simulink model "Leader"  (R2024b)
settings: Solver=ode4  StartTime=0  StopTime=100  FixedStep=0.001  RelTol=1e-3
undefined symbols (not defined in the file or in its folder): DiscIntNeverNeededParam
libraries: simulink x22, vrlib x1
(part 1 of 4)
settings Model: Creator=moham  LastModifiedBy=Omar
settings SolverCC: AlgebraicLoopSolver=TrustRegion
settings DataIOCC: ReturnWorkspaceOutputs=off
settings OptimizationCC: ReuseModelBlockBuffer=off
settings DebuggingCC: UnconnectedInputMsg=warning  UnconnectedOutputMsg=warning  UnconnectedLineMsg=warning  ArithmeticOperatorsInVariantConditions=warning
settings ModelReferenceCC: EnableRefExpFcnMdlSchedulingChecks=on
settings SFSimCC: SimUseLocalCustomCode=off  CustomCodeUndefinedFunction=UseInterfaceOnly
settings RTWCC: RTWUseLocalCustomCode=off  GPUComputeCapability=3.5

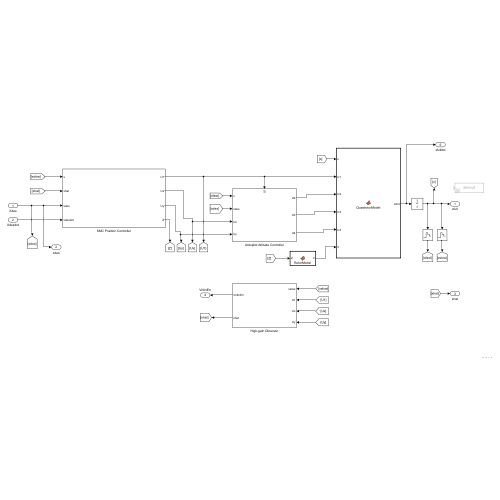
[thumbnail: Simulink's stored preview of the top-level diagram]
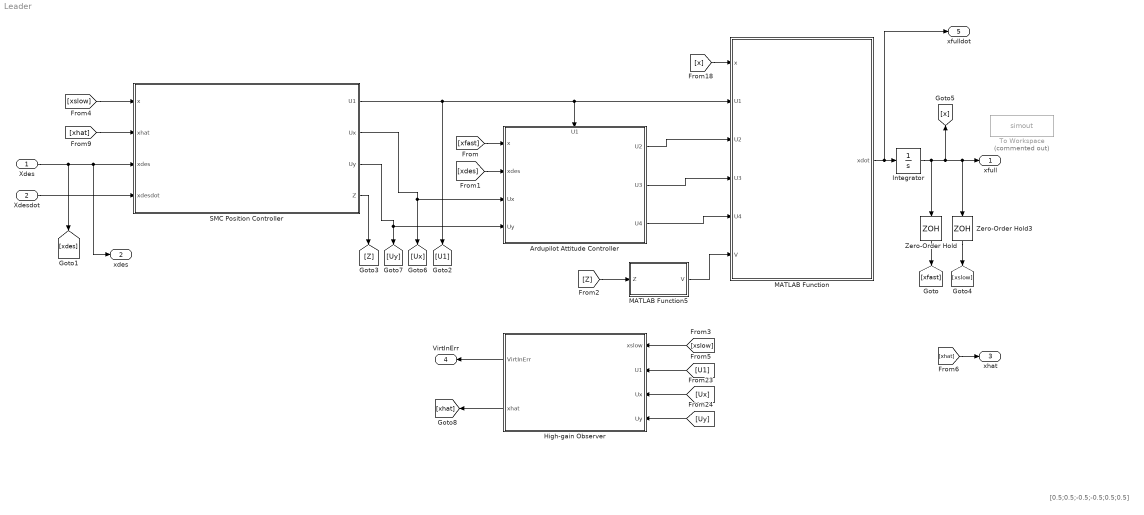
== system Leader ==
  note: [0.5;0.5;-0.5;-0.5;0.5;0.5]
  Xdes : Inport
  Xdesdot : Inport  Port=2  PortDimensions=12
  Ardupilot Attitude Controller : Subsystem
      settings: PortSchema="{\"entries\":[{\"content\":{\"sides\":[{\"content\":{\"connectorIds\":[\"In1\",\"In2\",\"In3\",\"In4\"]},\"type\":\"ConnectorPlacement.EquallySpacedRectSide\",\"uuid\":\"bad7bc7b-c5aa-4aa4-9de0-2ec046c1796f\"},{\"content\":{\"connectorIds\":[\"Out1\",\"Out2\",\"Out3\"],\"side\":\"RIGHT\"},\"type\":\"ConnectorPlacement.EquallySpacedRectSide\",\"uuid\":\"8bce01b0-d4dd-493d-8a35-b9dc86decf14\"},{\"content\":{\"connectorIds\":[\"In5\"],\"side\":\"TOP\"},\"type\":\"ConnectorPlacement.EquallySpacedRectSide\",\"uuid\":\"7d374ae2-e477-4008-a0c5-b6f4f89ed51f\"}]},\"type\":\"ConnectorPlacement.EquallySpacedConnector\",\"uuid\":\"7f04a3db-e2da-43c2-a92f-32b1947c5415\"}],\"packageUris\":[\"http://schema.mathworks.com/mf0/Connector/19700101\"],\"version\":\"1.0\"}"
  High-gain Observer : Subsystem
  Integrator : Integrator  InitialCondition=[0;0;0;0;0;0;0;0;0;0;0;0;0;0;0;0]
  MATLAB Function : MATLAB Function  TreatAsAtomicUnit=on
  MATLAB Function5 : MATLAB Function  TreatAsAtomicUnit=on
  SMC Position Controller : Subsystem
  To Workspace : ToWorkspace  Commented=on  VariableName=simout  SampleTime=-1
  Zero-Order Hold : ZeroOrderHold  SampleTime=0.01
  Zero-Order Hold3 : ZeroOrderHold  SampleTime=0.02
  xfull : Outport  VectorParamsAs1DForOutWhenUnconnected=off
  xdes : Outport  Port=2  VectorParamsAs1DForOutWhenUnconnected=off
  xhat : Outport  Port=3
  VirtInErr : Outport  Port=4
  xfulldot : Outport  Port=5
  wires:
  MATLAB Function5/1(V) -> MATLAB Function/6(V)
  MATLAB Function/1(xdot) -> xfulldot/1, Integrator/1
  Integrator/1 -> Zero-Order Hold3/1, xfull/1, [x], Zero-Order Hold/1
  Ardupilot Attitude Controller/1(U2) -> MATLAB Function/3(U2)
  Ardupilot Attitude Controller/2(U3) -> MATLAB Function/4(U3)
  Ardupilot Attitude Controller/3(U4) -> MATLAB Function/5(U4)
  [xdes] -> Ardupilot Attitude Controller/2(xdes)
  [x] -> MATLAB Function/1(x)
  [xslow] -> SMC Position Controller/1(x)
  [xhat] -> SMC Position Controller/2(xhat)
  Xdes/1 -> SMC Position Controller/3(xdes), xdes/1, [xdes]
  Xdesdot/1 -> SMC Position Controller/4(xdesdot)
  SMC Position Controller/1(U1) -> Ardupilot Attitude Controller/5(U1), MATLAB Function/2(U1), [U1]
  SMC Position Controller/2(Ux) -> [Ux], Ardupilot Attitude Controller/3(Ux)
  SMC Position Controller/3(Uy) -> Ardupilot Attitude Controller/4(Uy), [Uy]
  SMC Position Controller/4(Z) -> [Z]
  [Z] -> MATLAB Function5/1(Z)
  Zero-Order Hold/1 -> [xfast]
  Zero-Order Hold3/1 -> [xslow]
  [xhat] -> xhat/1
  [xfast] -> Ardupilot Attitude Controller/1(x)
  [U1] -> High-gain Observer/2(U1)
  [Ux] -> High-gain Observer/3(Ux)
  [Uy] -> High-gain Observer/4(Uy)
  [xslow] -> High-gain Observer/1(xslow)
  High-gain Observer/2(xhat) -> [xhat]
  High-gain Observer/1(VirtInErr) -> VirtInErr/1

== system Leader/Ardupilot Attitude Controller ==
  note: Get Desired Attitude
  note: Forward Desired Yaw and Convert: Virtual
      | Inputs --> Desired Roll and Pitch angles
  note: Rate Controller
  note: Attitude Controller
  x : Inport
  xdes : Inport  Port=2
  Ux : Inport  Port=3
  Uy : Inport  Port=4
  U1 : Inport  Port=5
  Attitude Controller : Subsystem
      settings: PortSchema="{\"entries\":[{\"content\":{\"sides\":[{\"content\":{\"connectorIds\":[\"In1\",\"In2\",\"In3\",\"In4\"]},\"type\":\"ConnectorPlacement.EquallySpacedRectSide\",\"uuid\":\"ec7fb444-4fa0-4c75-9921-499ce0d65b3a\"},{\"content\":{\"connectorIds\":[\"Out1\",\"Out2\",\"Out3\",\"Out4\"],\"side\":\"RIGHT\"},\"type\":\"ConnectorPlacement.EquallySpacedRectSide\",\"uuid\":\"c514eb8b-c928-4fdc-8f94-1e92d461987d\"},{\"content\":{\"connectorIds\":[],\"side\":\"TOP\"},\"type\":\"ConnectorPlacement.EquallySpacedRectSide\",\"uuid\":\"c9522f68-fcfa-40bc-963d-dafc938ce27d\"},{\"content\":{\"connectorIds\":[\"In5\",\"In6\",\"In7\"],\"side\":\"BOTTOM\"},\"type\":\"ConnectorPlacement.EquallySpacedRectSide\",\"uuid\":\"bc7d5f1e-3200-477e-805f-b3259f0159e2\"}]},\"type\":\"ConnectorPlacement.EquallySpacedConnector\",\"uuid\":\"993ff006-2c19-4b52-a807-2d91f7e143b6\"}],\"packageUris\":[\"http://schema.mathworks.com/mf0/Connector/19700101\"],\"version\":\"1.0\"}"
  Demux : Demux  Outputs=3
  Divide : Product  Inputs=*/
  MATLAB Function : MATLAB Function  TreatAsAtomicUnit=on
  MATLAB Function4 : MATLAB Function
  Max Thrust : Constant  Value=39
  Rate Controller : Subsystem
      settings: PortSchema="{\"entries\":[{\"content\":{\"sides\":[{\"content\":{\"connectorIds\":[\"In1\",\"In2\",\"In3\"]},\"type\":\"ConnectorPlacement.EquallySpacedRectSide\",\"uuid\":\"8a701ca7-ce38-496e-9f89-73a8426d5a34\"},{\"content\":{\"connectorIds\":[\"Out1\",\"Out2\",\"Out3\"],\"side\":\"RIGHT\"},\"type\":\"ConnectorPlacement.EquallySpacedRectSide\",\"uuid\":\"363a0e2e-6acc-4f21-9121-ba7c8748d9b4\"},{\"content\":{\"connectorIds\":[],\"side\":\"TOP\"},\"type\":\"ConnectorPlacement.EquallySpacedRectSide\",\"uuid\":\"4d7a2121-90ee-4dbe-91e3-b86ad0b96fd9\"},{\"content\":{\"connectorIds\":[\"In4\",\"In5\",\"In6\"],\"side\":\"BOTTOM\"},\"type\":\"ConnectorPlacement.EquallySpacedRectSide\",\"uuid\":\"495eef18-c57e-4f49-baa4-5500712935f3\"}]},\"type\":\"ConnectorPlacement.EquallySpacedConnector\",\"uuid\":\"9c8722b4-18d5-4647-94e4-af7446d3f664\"}],\"packageUris\":[\"http://schema.mathworks.com/mf0/Connector/19700101\"],\"version\":\"1.0\"}"
  Scope3 : Scope  NumInputPorts=3
  Selector2 : Selector  InputPortWidth=16  IndexOptions=Index vector (dialog)  Indices=[1 3 5]  OutputSizes=1
  Selector3 : Selector  InputPortWidth=16  IndexOptions=Index vector (dialog)  Indices=[2 4 6]  OutputSizes=1
  Terminator : Terminator
  U2 : Outport  VectorParamsAs1DForOutWhenUnconnected=off
  U3 : Outport  Port=2  VectorParamsAs1DForOutWhenUnconnected=off
  U4 : Outport  Port=3  VectorParamsAs1DForOutWhenUnconnected=off
  wires:
  xdes/1 -> MATLAB Function4/2(xdes)
  Attitude Controller/1(rollRateTar) -> Rate Controller/1(rollRateDes)  "rollRateTar"
  Attitude Controller/4(feedforwardScaler) -> Terminator/1
  Attitude Controller/2(pitchRateTar) -> Rate Controller/2(pitchRateDes)  "pitchRateTar"
  Attitude Controller/3(yawRateTar) -> Rate Controller/3(yawRateDes)  "yawRateTar"
  x/1 -> MATLAB Function4/1(x), [x]
  Max Thrust/1 -> Divide/2
  Divide/1 -> [throttle]
  [throttle] -> Attitude Controller/1(throttle)
  MATLAB Function4/1(phi_des) -> Attitude Controller/2(rollAngDes)
  MATLAB Function4/2(theta_des) -> Attitude Controller/3(pitchAngDes)
  MATLAB Function4/3(psidot_des) -> Attitude Controller/4(yawRateDes)
  [x] -> Selector3/1, Selector2/1
  Selector2/1 -> [eulerAct]
  Selector3/1 -> [ratesAct]
  [eulerAct] -> MATLAB Function/1(euler), Attitude Controller/5(eulerAngleAct)
  MATLAB Function/1(q) -> Attitude Controller/6(attitudeBodyAct)
  [ratesAct] -> Attitude Controller/7(angRatesBf)
  Demux/1 -> Rate Controller/4(rollRateAct)
  Demux/2 -> Rate Controller/5(pitchRateAct)
  Demux/3 -> Rate Controller/6(yawRateAct)
  Rate Controller/1(rollRateCtrlOut) -> U2/1, Scope3/1
  Rate Controller/2(pitchRateCtrlOut) -> Scope3/2, U3/1
  Rate Controller/3(yawRateCtrlOut) -> Scope3/3, U4/1
  Ux/1 -> MATLAB Function4/3(Ux)
  Uy/1 -> MATLAB Function4/4(Uy)
  U1/1 -> Divide/1
  [ratesAct] -> Demux/1

== system Leader/High-gain Observer ==
  note: Inputs
  note: Trapezoidal Integration for
      | Estimation Errors in Z
  note: High-gain Observer
      | (Updating State Estimates)
  note: Outputs
  xslow : Inport
  U1 : Inport  Port=2
  Ux : Inport  Port=3
  Uy : Inport  Port=4
  Discrete-Time Integrator : DiscreteIntegrator  SampleTime=-1  ICPrevOutput=DiscIntNeverNeededParam  ICPrevScaledInput=DiscIntNeverNeededParam
  Integrator1 : Integrator  InitialCondition=[0.0;0.0;-1;0;0;0]
  MATLAB Function2 : MATLAB Function  TreatAsAtomicUnit=on
  Mux1 : Mux  Inputs=2
  Selector : Selector  InputPortWidth=16  IndexOptions=Index vector (dialog)  Indices=[11]  OutputSizes=1
  Selector1 : Selector  InputPortWidth=6  IndexOptions=Index vector (dialog)  Indices=[5]  OutputSizes=1
  Sum : Sum  Inputs=|+-
  Sum1 : Sum  Inputs=|+-
  Zero-Order Hold2 : ZeroOrderHold  SampleTime=0.02
  VirtInErr : Outport
  xhat : Outport  Port=2
  wires:
  Zero-Order Hold2/1 -> [xhat]
  Mux1/1 -> Sum1/2
  [xslow] -> MATLAB Function2/1(x)
  MATLAB Function2/2(UxUyact) -> Sum1/1
  [xhat] -> Selector1/1
  MATLAB Function2/1(xhatdot) -> Integrator1/1
  [Ux] -> Mux1/1
  [U1] -> MATLAB Function2/4(U1)
  Integrator1/1 -> Zero-Order Hold2/1
  Sum1/1 -> VirtInErr/1
  [Uy] -> Mux1/2
  Sum/1 -> Discrete-Time Integrator/1
  [xhat] -> MATLAB Function2/3(xhat)
  Selector/1 -> Sum/1
  Selector1/1 -> Sum/2
  U1/1 -> [U1]
  Ux/1 -> [Ux]
  Uy/1 -> [Uy]
  xslow/1 -> [xslow]
  [xslow] -> Selector/1
  Discrete-Time Integrator/1 -> MATLAB Function2/2(zintg)
  [xhat] -> xhat/1

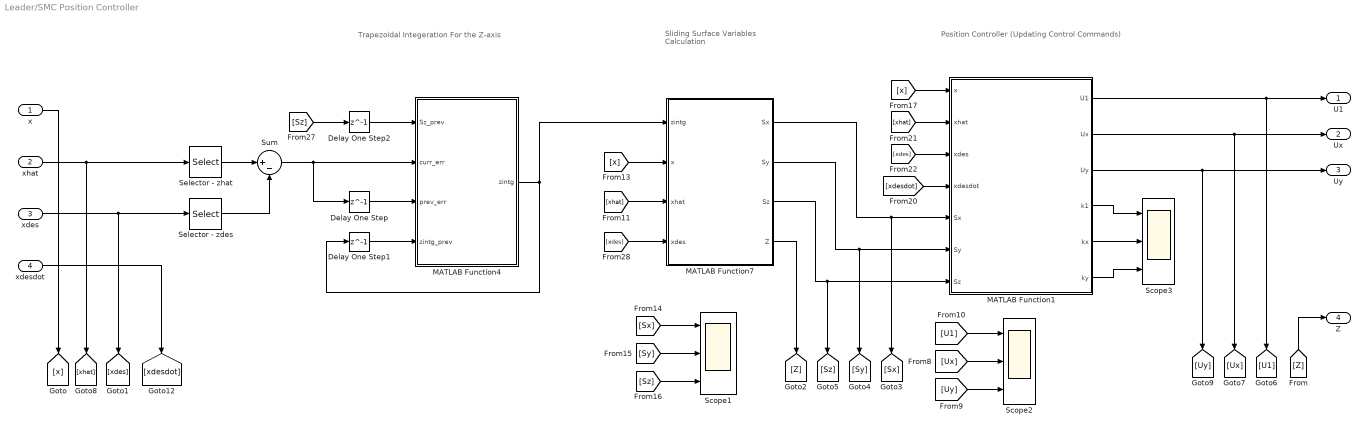
== system Leader/SMC Position Controller ==
  note: Sliding Surface
      | Variables Calculation
  note: Trapezoidal Integeration
      | For the Z-axis
  note: Position Controller
      | (Updating Control Commands)
  x : Inport
  xhat : Inport  Port=2
  xdes : Inport  Port=3
  xdesdot : Inport  Port=4
  Delay One Step : Delay  DelayLength=1
  Delay One Step1 : Delay  DelayLength=1
  Delay One Step2 : Delay  DelayLength=1
  MATLAB Function1 : MATLAB Function  TreatAsAtomicUnit=on
  MATLAB Function4 : MATLAB Function  TreatAsAtomicUnit=on
  MATLAB Function7 : MATLAB Function  TreatAsAtomicUnit=on
  Scope1 : Scope  NumInputPorts=3
  Scope2 : Scope  NumInputPorts=3
  Scope3 : Scope  NumInputPorts=3
  Selector - zdes : Selector  InputPortWidth=12  IndexOptions=Index vector (dialog)  Indices=[11]  OutputSizes=1
  Selector - zhat : Selector  InputPortWidth=6  IndexOptions=Index vector (dialog)  Indices=[5]  OutputSizes=1
  Sum : Sum  Inputs=|+-
  U1 : Outport
  Ux : Outport  Port=2
  Uy : Outport  Port=3
  Z : Outport  Port=4
  wires:
  [Sz] -> Delay One Step2/1
  Selector - zhat/1 -> Sum/1
  Sum/1 -> Delay One Step/1, MATLAB Function4/2(curr_err)
  Delay One Step2/1 -> MATLAB Function4/1(Sz_prev)
  Delay One Step1/1 -> MATLAB Function4/4(zintg_prev)
  MATLAB Function4/1(zintg) -> MATLAB Function7/1(zintg), Delay One Step1/1
  Selector - zdes/1 -> Sum/2
  Delay One Step/1 -> MATLAB Function4/3(prev_err)
  xhat/1 -> [xhat], Selector - zhat/1
  xdes/1 -> [xdes], Selector - zdes/1
  [xdes] -> MATLAB Function7/4(xdes)
  [xhat] -> MATLAB Function7/3(xhat)
  [x] -> MATLAB Function7/2(x)
  x/1 -> [x]
  xdesdot/1 -> [xdesdot]
  [xdesdot] -> MATLAB Function1/4(xdesdot)
  [x] -> MATLAB Function1/1(x)
  [xhat] -> MATLAB Function1/2(xhat)
  [xdes] -> MATLAB Function1/3(xdes)
  MATLAB Function7/1(Sx) -> [Sx], MATLAB Function1/5(Sx)
  MATLAB Function7/2(Sy) -> [Sy], MATLAB Function1/6(Sy)
  MATLAB Function7/3(Sz) -> [Sz], MATLAB Function1/7(Sz)
  MATLAB Function7/4(Z) -> [Z]
  MATLAB Function1/1(U1) -> [U1], U1/1
  MATLAB Function1/2(Ux) -> [Ux], Ux/1
  MATLAB Function1/3(Uy) -> [Uy], Uy/1
  [Z] -> Z/1
  [Sz] -> Scope1/3
  [U1] -> Scope2/1
  [Sy] -> Scope1/2
  [Sx] -> Scope1/1
  [Ux] -> Scope2/2
  [Uy] -> Scope2/3
  MATLAB Function1/4(k1) -> Scope3/1
  MATLAB Function1/5(kx) -> Scope3/2
  MATLAB Function1/6(ky) -> Scope3/3

== system Leader/Ardupilot Attitude Controller/Attitude Controller ==
  note: input_euler_angle_roll_pitch_euler_rate_yaw() & attitude_controller_run_quat()
      | Calculation of target euler rates and angles and angular velocities
  note: Sponsored by IAV GmbH
  throttle : Inport
  rollAngDes : Inport  Port=2
  pitchAngDes : Inport  Port=3
  yawRateDes : Inport  Port=4
  eulerAngleAct : Inport  Port=5
  attitudeBodyAct : Inport  Port=6
  angRatesBf : Inport  Port=7
  Demux : Demux  Outputs=3
  input_euler_angle_roll_pitch_euler_rate_yaw() : Subsystem
  rollRateTar : Outport
  pitchRateTar : Outport  Port=2
  yawRateTar : Outport  Port=3
  feedforwardScaler : Outport  Port=4
  wires:
  attitudeBodyAct/1 -> input_euler_angle_roll_pitch_euler_rate_yaw()/6(attitudeBodyAct)
  angRatesBf/1 -> input_euler_angle_roll_pitch_euler_rate_yaw()/7(angRatesBf)
  Demux/2 -> pitchRateTar/1
  Demux/1 -> rollRateTar/1
  Demux/3 -> yawRateTar/1
  input_euler_angle_roll_pitch_euler_rate_yaw()/1(angVelBodyTarget) -> Demux/1  "angVelBody"
  input_euler_angle_roll_pitch_euler_rate_yaw()/2(feedforwardScaler) -> feedforwardScaler/1
  eulerAngleAct/1 -> input_euler_angle_roll_pitch_euler_rate_yaw()/5(eulerAngleAct)
  throttle/1 -> input_euler_angle_roll_pitch_euler_rate_yaw()/1(throttle)
  rollAngDes/1 -> input_euler_angle_roll_pitch_euler_rate_yaw()/2(rollAngDes)
  pitchAngDes/1 -> input_euler_angle_roll_pitch_euler_rate_yaw()/3(pitchAngDes)
  yawRateDes/1 -> input_euler_angle_roll_pitch_euler_rate_yaw()/4(yawRateDes)

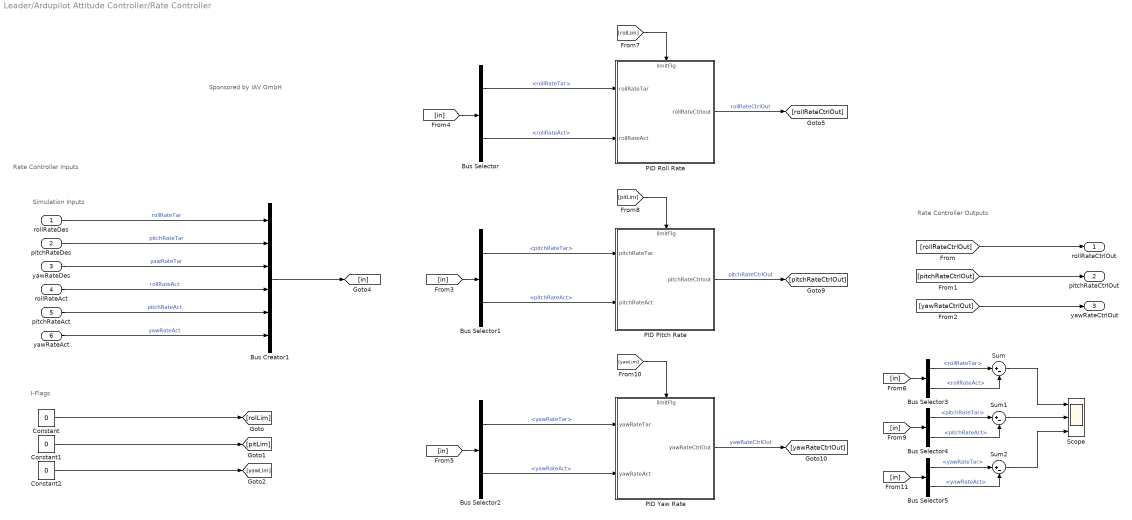
== system Leader/Ardupilot Attitude Controller/Rate Controller ==
  note: I-Flags
  note: Rate Controller Inputs
  note: Rate Controller Outputs
  note: Simulation Inputs
  note: Sponsored by IAV GmbH
  rollRateDes : Inport
  pitchRateDes : Inport  Port=2
  yawRateDes : Inport  Port=3
  rollRateAct : Inport  Port=4
  pitchRateAct : Inport  Port=5
  yawRateAct : Inport  Port=6
  Bus Creator1 : BusCreator  Inputs=6
  Bus Selector : BusSelector  OutputSignals=rollRateTar,rollRateAct
  Bus Selector1 : BusSelector  OutputSignals=pitchRateTar,pitchRateAct
  Bus Selector2 : BusSelector  OutputSignals=yawRateTar,yawRateAct
  Bus Selector3 : BusSelector  OutputSignals=rollRateTar,rollRateAct
  Bus Selector4 : BusSelector  OutputSignals=pitchRateTar,pitchRateAct
  Bus Selector5 : BusSelector  OutputSignals=yawRateTar,yawRateAct
  Constant : Constant  Value=0
  Constant1 : Constant  Value=0
  Constant2 : Constant  Value=0
  PID Pitch Rate : Subsystem
      settings: PortSchema="{\"entries\":[{\"content\":{\"sides\":[{\"content\":{\"connectorIds\":[\"In1\",\"In2\"]},\"type\":\"ConnectorPlacement.EquallySpacedRectSide\",\"uuid\":\"c953bf57-30fb-4394-aa81-6fda736b57a6\"},{\"content\":{\"connectorIds\":[\"Out1\"],\"side\":\"RIGHT\"},\"type\":\"ConnectorPlacement.EquallySpacedRectSide\",\"uuid\":\"3c7ad81e-0863-4191-b28a-a9c07f820a0a\"},{\"content\":{\"connectorIds\":[\"In3\"],\"side\":\"TOP\"},\"type\":\"ConnectorPlacement.EquallySpacedRectSide\",\"uuid\":\"d279fa4b-d6e6-48af-a4f1-9d8595a6d70c\"}]},\"type\":\"ConnectorPlacement.EquallySpacedConnector\",\"uuid\":\"40596868-642f-4372-b8bb-11353e7a9cdb\"}],\"packageUris\":[\"http://schema.mathworks.com/mf0/Connector/19700101\"],\"version\":\"1.0\"}"
  PID Roll Rate : Subsystem
      settings: PortSchema="{\"entries\":[{\"content\":{\"sides\":[{\"content\":{\"connectorIds\":[\"In1\",\"In2\"]},\"type\":\"ConnectorPlacement.EquallySpacedRectSide\",\"uuid\":\"ccc00f8c-3713-4b46-9b2d-67fda6f44eb9\"},{\"content\":{\"connectorIds\":[\"Out1\"],\"side\":\"RIGHT\"},\"type\":\"ConnectorPlacement.EquallySpacedRectSide\",\"uuid\":\"24a560ef-4b0d-44d4-b17e-8cb38dfcb6b4\"},{\"content\":{\"connectorIds\":[\"In3\"],\"side\":\"TOP\"},\"type\":\"ConnectorPlacement.EquallySpacedRectSide\",\"uuid\":\"cd43f1cb-999b-4e44-9f37-57514624398c\"}]},\"type\":\"ConnectorPlacement.EquallySpacedConnector\",\"uuid\":\"35b9a70d-95bd-44f6-87a8-68a113e8ff9b\"}],\"packageUris\":[\"http://schema.mathworks.com/mf0/Connector/19700101\"],\"version\":\"1.0\"}"
  PID Yaw Rate : Subsystem
      settings: PortSchema="{\"entries\":[{\"content\":{\"sides\":[{\"content\":{\"connectorIds\":[\"In1\",\"In2\"]},\"type\":\"ConnectorPlacement.EquallySpacedRectSide\",\"uuid\":\"e641bc52-3ba8-4abf-91e5-f3e8f1d63eab\"},{\"content\":{\"connectorIds\":[\"Out1\"],\"side\":\"RIGHT\"},\"type\":\"ConnectorPlacement.EquallySpacedRectSide\",\"uuid\":\"7d55638e-b8f2-47ab-a11f-a4e45a3d6a7b\"},{\"content\":{\"connectorIds\":[\"In3\"],\"side\":\"TOP\"},\"type\":\"ConnectorPlacement.EquallySpacedRectSide\",\"uuid\":\"6a487507-9fdf-4d3e-b86b-b3f94c6d2850\"}]},\"type\":\"ConnectorPlacement.EquallySpacedConnector\",\"uuid\":\"38d20622-e21d-450d-bf23-0a2964a9c200\"}],\"packageUris\":[\"http://schema.mathworks.com/mf0/Connector/19700101\"],\"version\":\"1.0\"}"
  Scope : Scope  NumInputPorts=3
  Sum : Sum  Inputs=|+-
  Sum1 : Sum  Inputs=|+-
  Sum2 : Sum  Inputs=|+-
  rollRateCtrlOut : Outport
  pitchRateCtrlOut : Outport  Port=2
  yawRateCtrlOut : Outport  Port=3
  wires:
  PID Yaw Rate/1(yawRateCtrlOut) -> [yawRateCtrlOut]  "yawRateCtrlOut"
  Bus Selector/1 -> PID Roll Rate/1(rollRateTar)  "<rollRateTar>"
  Bus Selector/2 -> PID Roll Rate/2(rollRateAct)  "<rollRateAct>"
  Bus Selector2/1 -> PID Yaw Rate/1(yawRateTar)  "<yawRateTar>"
  PID Pitch Rate/1(pitchRateCtrlout) -> [pitchRateCtrlOut]  "pitchRateCtrlOut"
  Bus Selector2/2 -> PID Yaw Rate/2(yawRateAct)  "<yawRateAct>"
  PID Roll Rate/1(rollRateCtrlout) -> [rollRateCtrlOut]  "rollRateCtrlOut"
  [rollRateCtrlOut] -> rollRateCtrlOut/1
  [pitchRateCtrlOut] -> pitchRateCtrlOut/1
  [yawRateCtrlOut] -> yawRateCtrlOut/1
  rollRateAct/1 -> Bus Creator1/4  "rollRateAct"
  pitchRateAct/1 -> Bus Creator1/5  "pitchRateAct"
  yawRateAct/1 -> Bus Creator1/6  "yawRateAct"
  yawRateDes/1 -> Bus Creator1/3  "yawRateTar"
  pitchRateDes/1 -> Bus Creator1/2  "pitchRateTar"
  rollRateDes/1 -> Bus Creator1/1  "rollRateTar"
  Bus Creator1/1 -> [in]
  [in] -> Bus Selector/1
  [in] -> Bus Selector1/1
  [in] -> Bus Selector2/1
  Bus Selector1/1 -> PID Pitch Rate/1(pitchRateTar)  "<pitchRateTar>"
  Bus Selector1/2 -> PID Pitch Rate/2(pitchRateAct)  "<pitchRateAct>"
  Constant/1 -> [rolLim]
  Constant1/1 -> [pitLim]
  Constant2/1 -> [yawLim]
  [rolLim] -> PID Roll Rate/3(limitFlg)
  [pitLim] -> PID Pitch Rate/3(limitFlg)
  [yawLim] -> PID Yaw Rate/3(limitFlg)
  [in] -> Bus Selector3/1
  Bus Selector3/1 -> Sum/1  "<rollRateTar>"
  Bus Selector3/2 -> Sum/2  "<rollRateAct>"
  Bus Selector4/2 -> Sum1/2  "<pitchRateAct>"
  Bus Selector4/1 -> Sum1/1  "<pitchRateTar>"
  [in] -> Bus Selector4/1
  Bus Selector5/2 -> Sum2/2  "<yawRateAct>"
  Bus Selector5/1 -> Sum2/1  "<yawRateTar>"
  [in] -> Bus Selector5/1
  Sum1/1 -> Scope/2
  Sum/1 -> Scope/1
  Sum2/1 -> Scope/3

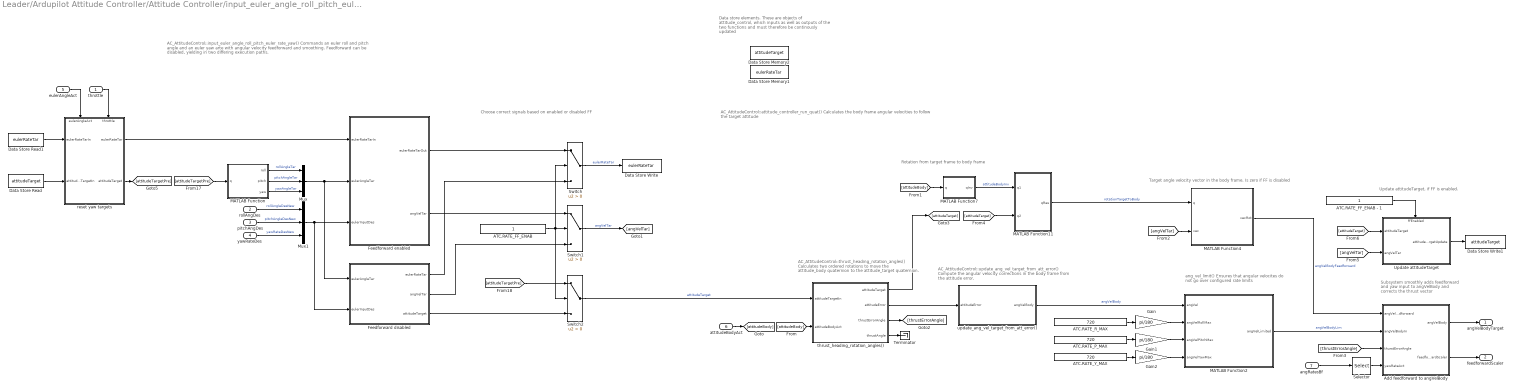
== system Leader/Ardupilot Attitude Controller/Attitude Controller/input_euler_angle_roll_pitch_euler_rate_yaw() ==
  note: Data store elements. These are objects of attitude_control, which inputs as well as outputs of the two functions and must therefore be continously updated
  note: Update attitudeTarget, if FF is enabled.
  note: Subsystem smoothly adds feedforward and yaw input to angVelBody and corrects the thrust vector
  note: Target angle velocity vector in the body frame. Is zero if FF is disabled
  note: Rotation from target frame to body frame
  note: Choose correct signals based on enabled or disabled FF
  note: AC_AttitudeControl::input_euler_angle_roll_pitch_euler_rate_yaw()
      | Commands an euler roll and pitch angle and an euler yaw arte with angular velocity feedforward and smoothing.
      | Feedforward can be disabled, yielding in two differing execution paths.
  note: AC_AttitudeControl::thrust_heading_rotation_angles()
      | Calculates two ordered rotations to move the attitude_body quaternion to the attitude_target quaternion.
  note: AC_AttitudeControl::update_ang_vel_target_from_att_error()
      | Compute the angular velocity corrections in the body frame from the attitude error.
  note: ang_vel_limit()
      | Ensures that angular velocites do not go over configured rate limits
  note: AC_AttitudeControl::attitude_controller_run_quat()
      | Calculates the body frame angular velocities to follow the target attitude
  throttle : Inport
  rollAngDes : Inport  Port=2
  pitchAngDes : Inport  Port=3
  yawRateDes : Inport  Port=4
  eulerAngleAct : Inport  Port=5
  attitudeBodyAct : Inport  Port=6
  angRatesBf : Inport  Port=7
  ATC.RATE_FF_ENAB : Constant
  ATC.RATE_FF_ENAB - 1 : Constant
  ATC.RATE_P_MAX : Constant  Value=720
  ATC.RATE_R_MAX : Constant  Value=720
  ATC.RATE_Y_MAX : Constant  Value=720
  Add feedforward to angVelBody : Subsystem
  Data Store Memory1 : DataStoreMemory  DataStoreName=eulerRateTar  WriteAfterWriteMsg=warning  InitialValue=[0;0;0]  ShowAdditionalParam=off  OutDataTypeStr=double
  Data Store Memory2 : DataStoreMemory  DataStoreName=attitudeTarget  WriteAfterWriteMsg=warning  InitialValue=[1;0;0;0]  ShowAdditionalParam=off  OutDataTypeStr=double
  Data Store Read : DataStoreRead  DataStoreName=attitudeTarget  IndexOptions=Index vector (dialog)  Indices=1  OutputSizes=1
  Data Store Read1 : DataStoreRead  DataStoreName=eulerRateTar  IndexOptions=Index vector (dialog)  Indices=1  OutputSizes=1
  Data Store Write : DataStoreWrite  DataStoreName=eulerRateTar  IndexOptions=Index vector (dialog)  Indices=1  OutputSizes=1
  Data Store Write1 : DataStoreWrite  DataStoreName=attitudeTarget  IndexOptions=Index vector (dialog)  Indices=1  OutputSizes=1
  Feedforward disabled : Subsystem
  Feedforward enabled : Subsystem
  Gain : Gain  Gain=pi/180
  Gain1 : Gain  Gain=pi/180
  Gain2 : Gain  Gain=pi/180
  MATLAB Function : MATLAB Function  TreatAsAtomicUnit=on
  MATLAB Function11 : MATLAB Function  TreatAsAtomicUnit=on
  MATLAB Function2 : MATLAB Function  TreatAsAtomicUnit=on
  MATLAB Function4 : MATLAB Function  TreatAsAtomicUnit=on
  MATLAB Function7 : MATLAB Function  TreatAsAtomicUnit=on
  Mux : Mux  Inputs=3
  Mux1 : Mux  Inputs=3
  Selector : Selector  InputPortWidth=3  IndexOptions=Index vector (dialog)  Indices=[3]  OutputSizes=1
  Switch : Switch  Criteria=u2 > Threshold  SaturateOnIntegerOverflow=off  InputSameDT=off
  Switch1 : Switch  Criteria=u2 > Threshold  SaturateOnIntegerOverflow=off  InputSameDT=off
  Switch2 : Switch  Criteria=u2 > Threshold  SaturateOnIntegerOverflow=off  InputSameDT=off
  Terminator : Terminator
  Update attitudeTarget : Subsystem
      settings: PortSchema="{\"entries\":[{\"content\":{\"sides\":[{\"content\":{\"connectorIds\":[\"In1\",\"In2\"]},\"type\":\"ConnectorPlacement.EquallySpacedRectSide\",\"uuid\":\"677f2474-a933-4351-a18c-d191f7c74006\"},{\"content\":{\"connectorIds\":[\"Out1\"],\"side\":\"RIGHT\"},\"type\":\"ConnectorPlacement.EquallySpacedRectSide\",\"uuid\":\"e9b9097f-3644-4a9a-8149-04c97bd90a0c\"},{\"content\":{\"connectorIds\":[\"In3\"],\"side\":\"TOP\"},\"type\":\"ConnectorPlacement.EquallySpacedRectSide\",\"uuid\":\"2b4d5a13-4fc6-40d8-be4c-f1f4571d6c96\"}]},\"type\":\"ConnectorPlacement.EquallySpacedConnector\",\"uuid\":\"62980eaf-3b78-41ff-aa7a-c4a8a9508ced\"}],\"packageUris\":[\"http://schema.mathworks.com/mf0/Connector/R2020b\"],\"version\":\"1.0\"}"
  reset yaw targets : Subsystem
      settings: PortSchema="{\"entries\":[{\"content\":{\"sides\":[{\"content\":{\"connectorIds\":[\"In1\",\"In2\"]},\"type\":\"ConnectorPlacement.EquallySpacedRectSide\",\"uuid\":\"29284c76-4388-4ab2-b640-2aa249641a5e\"},{\"content\":{\"connectorIds\":[\"Out1\",\"Out2\"],\"side\":\"RIGHT\"},\"type\":\"ConnectorPlacement.EquallySpacedRectSide\",\"uuid\":\"b3687b33-33ad-4cf1-ba70-eea9295fb5e4\"},{\"content\":{\"connectorIds\":[\"In3\",\"In4\"],\"side\":\"TOP\"},\"type\":\"ConnectorPlacement.EquallySpacedRectSide\",\"uuid\":\"b547cb73-472d-403b-8f7c-c78a9fbe5228\"}]},\"type\":\"ConnectorPlacement.EquallySpacedConnector\",\"uuid\":\"31dffed6-fd3b-4288-90b3-a2b7b520dc2f\"}],\"packageUris\":[\"http://schema.mathworks.com/mf0/Connector/R2020b\"],\"version\":\"1.0\"}"
  thrust_heading_rotation_angles() : Subsystem
  update_ang_vel_target_from_att_error() : Subsystem
  angVelBodyTarget : Outport
  feedforwardScaler : Outport  Port=2
  wires:
  MATLAB Function/3(yaw) -> Mux/3  "yawAngleTar"
  MATLAB Function/2(pitch) -> Mux/2  "pitchAngleTar"
  MATLAB Function/1(roll) -> Mux/1  "rollAngleTar"
  Mux/1 -> Feedforward disabled/1(eulerAngleTar), Feedforward enabled/2(eulerAngleTar)
  rollAngDes/1 -> Mux1/1  "rollAngleDesNew"
  pitchAngDes/1 -> Mux1/2  "pitchAngleDesNew"
  yawRateDes/1 -> Mux1/3  "yawRateDesNew"
  Mux1/1 -> Feedforward enabled/3(eulerInputDes), Feedforward disabled/2(eulerInputDes)
  Data Store Read1/1 -> reset yaw targets/1(eulerRateTarIn)
  Feedforward enabled/1(eulerRateTarOut) -> Switch/1
  Feedforward disabled/1(eulerRateTar) -> Switch/3
  Feedforward enabled/2(angVelTar) -> Switch1/1
  Feedforward disabled/2(angVelTar) -> Switch1/3
  Switch/1 -> Data Store Write/1  "eulerRateTar"
  Switch1/1 -> [angVelTar]  "angVelTar"
  ATC.RATE_FF_ENAB/1 -> Switch2/2, Switch/2, Switch1/2
  [attitudeTargetPre] -> Switch2/1
  Feedforward disabled/3(attitudeTarget) -> Switch2/3
  Switch2/1 -> thrust_heading_rotation_angles()/1(attitudeTargetIn)  "attitudeTarget"
  [attitudeBody] -> thrust_heading_rotation_angles()/2(attitudeBodyAct)
  thrust_heading_rotation_angles()/4(thrustAngle) -> Terminator/1
  thrust_heading_rotation_angles()/2(attitudeError) -> update_ang_vel_target_from_att_error()/1(attitudeError)
  ATC.RATE_P_MAX/1 -> Gain1/1
  ATC.RATE_R_MAX/1 -> Gain/1
  Gain2/1 -> MATLAB Function2/4(angVelYawMax)
  Gain1/1 -> MATLAB Function2/3(angVelPitchMax)
  ATC.RATE_Y_MAX/1 -> Gain2/1
  Gain/1 -> MATLAB Function2/2(angVelRollMax)
  update_ang_vel_target_from_att_error()/1(angVelBody) -> MATLAB Function2/1(angVel)  "angVelBody"
  attitudeBodyAct/1 -> [attitudeBody]
  thrust_heading_rotation_angles()/1(attitudeTarget) -> [attitudeTarget]
  [attitudeBody] -> MATLAB Function7/1(q)
  MATLAB Function7/1(qInv) -> MATLAB Function11/1(q1)  "attitudeBodyInv"
  MATLAB Function11/1(qRes) -> MATLAB Function4/1(q)  "rotationTargetToBody"
  [angVelTar] -> MATLAB Function4/2(vec)
  MATLAB Function4/1(vecRot) -> Add feedforward to angVelBody/1(angVelBodyFeedforward)  "angVelBodyFeedforward"
  thrust_heading_rotation_angles()/3(thrustErrorAngle) -> [thrustErrorAngle]
  MATLAB Function2/1(angVelLimited) -> Add feedforward to angVelBody/2(angVelBodyIn)  "angVelBodyLim"
  [thrustErrorAngle] -> Add feedforward to angVelBody/3(thurstErrorAngle)
  angRatesBf/1 -> Selector/1
  Selector/1 -> Add feedforward to angVelBody/4(yawRateAct)
  [attitudeTarget] -> MATLAB Function11/2(q2)
  [angVelTar] -> Update attitudeTarget/2(angVelTar)
  Add feedforward to angVelBody/1(angVelBody) -> angVelBodyTarget/1
  [attitudeTarget] -> Update attitudeTarget/1(attitudeTarget)
  Update attitudeTarget/1(attitudeTargetUpdate) -> Data Store Write1/1
  ATC.RATE_FF_ENAB - 1/1 -> Update attitudeTarget/3(ffEnabled)
  Add feedforward to angVelBody/2(feedforwardScaler) -> feedforwardScaler/1
  Data Store Read/1 -> reset yaw targets/2(attitudeTargetIn)
  reset yaw targets/1(eulerRateTar) -> Feedforward enabled/1(eulerRateTarIn)
  eulerAngleAct/1 -> reset yaw targets/3(eulerAngleAct)
  [attitudeTargetPre] -> MATLAB Function/1(q)
  reset yaw targets/2(attitudeTarget) -> [attitudeTargetPre]
  throttle/1 -> reset yaw targets/4(throttle)

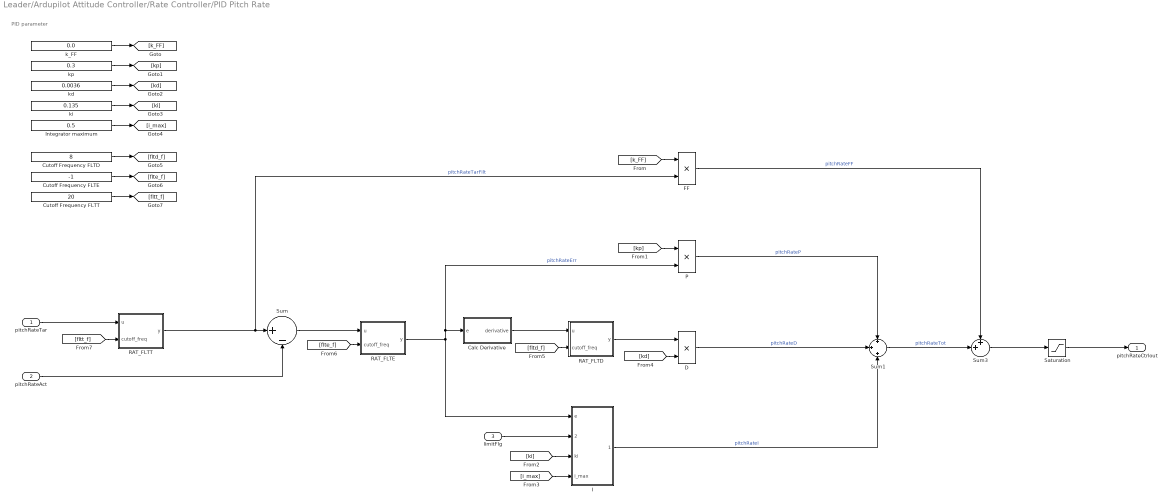
== system Leader/Ardupilot Attitude Controller/Rate Controller/PID Pitch Rate ==
  note: PID parameter
  pitchRateTar : Inport
  pitchRateAct : Inport  Port=2
  limitFlg : Inport  Port=3
  Calc Derivative : Subsystem
  Cutoff Frequency FLTD : Constant  Value=8
  Cutoff Frequency FLTE : Constant  Value=-1
  Cutoff Frequency FLTT : Constant  Value=20
  D : Product
  FF : Product
  I : Subsystem
  Integrator maximum : Constant  Value=0.5
  P : Product
  RAT_FLTD : Subsystem  TreatAsAtomicUnit=on
  RAT_FLTE : Subsystem  TreatAsAtomicUnit=on
  RAT_FLTT : Subsystem  TreatAsAtomicUnit=on
  Saturation : Saturate  UpperLimit=1.0  LowerLimit=-1.0
  Sum : Sum  Inputs=|+-
  Sum1 : Sum  Inputs=+|+|+
  Sum3 : Sum  Inputs=++|  OutDataTypeStr=double
  k_FF : Constant  Value=0.0
  kd : Constant  Value=0.0036
  ki : Constant  Value=0.135
  kp : Constant  Value=0.3
  pitchRateCtrlout : Outport
  wires:
  [flte_f] -> RAT_FLTE/2(cutoff_freq)
  Cutoff Frequency FLTT/1 -> [fltt_f]
  Cutoff Frequency FLTE/1 -> [flte_f]
  Cutoff Frequency FLTD/1 -> [fltd_f]
  Integrator maximum/1 -> [i_max]
  ki/1 -> [ki]
  kd/1 -> [kd]
  kp/1 -> [kp]
  k_FF/1 -> [k_FF]
  Sum/1 -> RAT_FLTE/1(u)
  pitchRateAct/1 -> Sum/2
  pitchRateTar/1 -> RAT_FLTT/1(u)
  RAT_FLTT/1(y) -> Sum/1, FF/2  "pitchRateTarFilt"
  Sum1/1 -> Sum3/2  "pitchRateTot"
  I/1(integrator) -> Sum1/3  "pitchRateI"
  D/1 -> Sum1/2  "pitchRateD"
  Calc Derivative/1(derivative) -> RAT_FLTD/1(u)
  P/1 -> Sum1/1  "pitchRateP"
  limitFlg/1 -> I/2(limitFlg)
  RAT_FLTE/1(y) -> I/1(e), Calc Derivative/1(e), P/2  "pitchRateErr"
  FF/1 -> Sum3/1  "pitchRateFF"
  [i_max] -> I/4(i_max)
  [fltd_f] -> RAT_FLTD/2(cutoff_freq)
  [k_FF] -> FF/1
  [kp] -> P/1
  [kd] -> D/2
  [ki] -> I/3(ki)
  [fltt_f] -> RAT_FLTT/2(cutoff_freq)
  RAT_FLTD/1(y) -> D/1
  Sum3/1 -> Saturation/1
  Saturation/1 -> pitchRateCtrlout/1

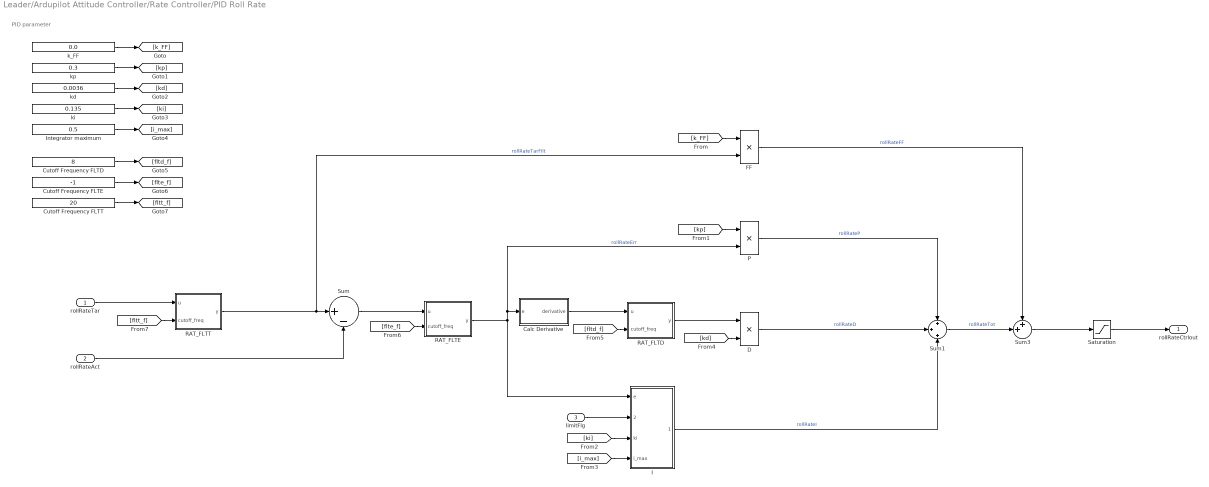
== system Leader/Ardupilot Attitude Controller/Rate Controller/PID Roll Rate ==
  note: PID parameter
  rollRateTar : Inport
  rollRateAct : Inport  Port=2
  limitFlg : Inport  Port=3
  Calc Derivative : Subsystem
  Cutoff Frequency FLTD : Constant  Value=8
  Cutoff Frequency FLTE : Constant  Value=-1
  Cutoff Frequency FLTT : Constant  Value=20
  D : Product
  FF : Product
  I : Subsystem
  Integrator maximum : Constant  Value=0.5
  P : Product
  RAT_FLTD : Subsystem  TreatAsAtomicUnit=on
  RAT_FLTE : Subsystem  TreatAsAtomicUnit=on
  RAT_FLTT : Subsystem  TreatAsAtomicUnit=on
  Saturation : Saturate  UpperLimit=1.0  LowerLimit=-1.0
  Sum : Sum  Inputs=|+-
  Sum1 : Sum  Inputs=+|+|+
  Sum3 : Sum  Inputs=++|  OutDataTypeStr=double
  k_FF : Constant  Value=0.0
  kd : Constant  Value=0.0036
  ki : Constant  Value=0.135
  kp : Constant  Value=0.3
  rollRateCtrlout : Outport
  wires:
  RAT_FLTE/1(y) -> P/2, Calc Derivative/1(e), I/1(e)  "rollRateErr"
  P/1 -> Sum1/1  "rollRateP"
  D/1 -> Sum1/2  "rollRateD"
  I/1(integrator) -> Sum1/3  "rollRateI"
  RAT_FLTT/1(y) -> FF/2, Sum/1  "rollRateTarFilt"
  rollRateTar/1 -> RAT_FLTT/1(u)
  rollRateAct/1 -> Sum/2
  Sum/1 -> RAT_FLTE/1(u)
  k_FF/1 -> [k_FF]
  kp/1 -> [kp]
  kd/1 -> [kd]
  ki/1 -> [ki]
  Integrator maximum/1 -> [i_max]
  Cutoff Frequency FLTD/1 -> [fltd_f]
  Cutoff Frequency FLTE/1 -> [flte_f]
  Cutoff Frequency FLTT/1 -> [fltt_f]
  [k_FF] -> FF/1
  [kp] -> P/1
  [ki] -> I/3(ki)
  [i_max] -> I/4(i_max)
  [kd] -> D/2
  [fltd_f] -> RAT_FLTD/2(cutoff_freq)
  [flte_f] -> RAT_FLTE/2(cutoff_freq)
  [fltt_f] -> RAT_FLTT/2(cutoff_freq)
  Sum1/1 -> Sum3/2  "rollRateTot"
  FF/1 -> Sum3/1  "rollRateFF"
  Calc Derivative/1(derivative) -> RAT_FLTD/1(u)
  limitFlg/1 -> I/2(limitFlg)
  RAT_FLTD/1(y) -> D/1
  Sum3/1 -> Saturation/1
  Saturation/1 -> rollRateCtrlout/1

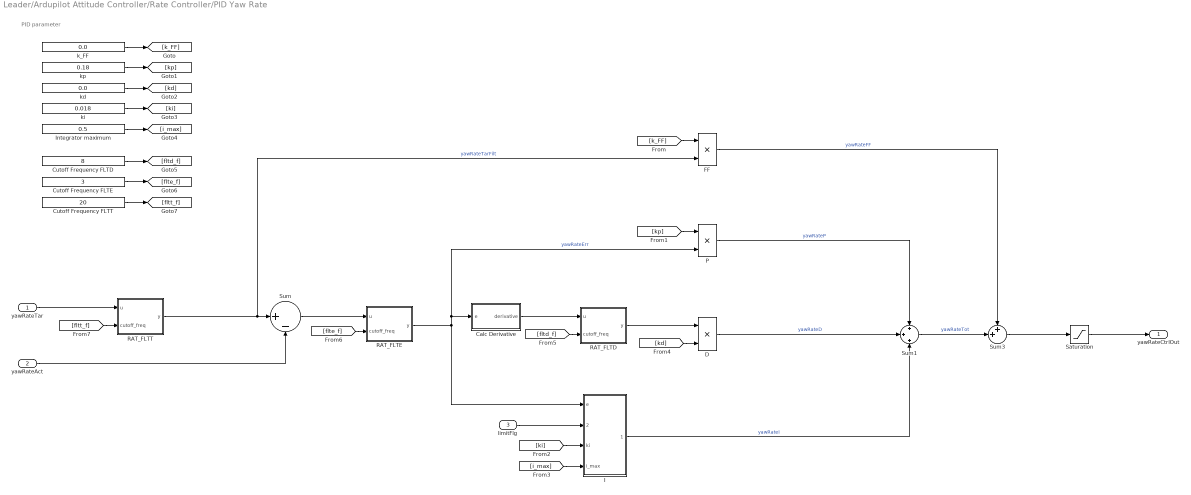
== system Leader/Ardupilot Attitude Controller/Rate Controller/PID Yaw Rate ==
  note: PID parameter
  yawRateTar : Inport
  yawRateAct : Inport  Port=2
  limitFlg : Inport  Port=3
  Calc Derivative : Subsystem
  Cutoff Frequency FLTD : Constant  Value=8
  Cutoff Frequency FLTE : Constant  Value=3
  Cutoff Frequency FLTT : Constant  Value=20
  D : Product
  FF : Product
  I : Subsystem
  Integrator maximum : Constant  Value=0.5
  P : Product
  RAT_FLTD : Subsystem  TreatAsAtomicUnit=on
  RAT_FLTE : Subsystem  TreatAsAtomicUnit=on
  RAT_FLTT : Subsystem  TreatAsAtomicUnit=on
  Saturation : Saturate  UpperLimit=1.0  LowerLimit=-1.0
  Sum : Sum  Inputs=|+-
  Sum1 : Sum  Inputs=+|+|+
  Sum3 : Sum  Inputs=++|  OutDataTypeStr=double
  k_FF : Constant  Value=0.0
  kd : Constant  Value=0.0
  ki : Constant  Value=0.018
  kp : Constant  Value=0.18
  yawRateCtrlOut : Outport
  wires:
  RAT_FLTE/1(y) -> I/1(e), Calc Derivative/1(e), P/2  "yawRateErr"
  limitFlg/1 -> I/2(limitFlg)
  P/1 -> Sum1/1  "yawRateP"
  Calc Derivative/1(derivative) -> RAT_FLTD/1(u)
  D/1 -> Sum1/2  "yawRateD"
  I/1(integrator) -> Sum1/3  "yawRateI"
  FF/1 -> Sum3/1  "yawRateFF"
  Sum1/1 -> Sum3/2  "yawRateTot"
  RAT_FLTT/1(y) -> FF/2, Sum/1  "yawRateTarFilt"
  yawRateTar/1 -> RAT_FLTT/1(u)
  yawRateAct/1 -> Sum/2
  Sum/1 -> RAT_FLTE/1(u)
  k_FF/1 -> [k_FF]
  kp/1 -> [kp]
  kd/1 -> [kd]
  ki/1 -> [ki]
  Integrator maximum/1 -> [i_max]
  Cutoff Frequency FLTD/1 -> [fltd_f]
  Cutoff Frequency FLTE/1 -> [flte_f]
  Cutoff Frequency FLTT/1 -> [fltt_f]
  [k_FF] -> FF/1
  [kp] -> P/1
  [ki] -> I/3(ki)
  [i_max] -> I/4(i_max)
  [kd] -> D/2
  [fltd_f] -> RAT_FLTD/2(cutoff_freq)
  [flte_f] -> RAT_FLTE/2(cutoff_freq)
  [fltt_f] -> RAT_FLTT/2(cutoff_freq)
  RAT_FLTD/1(y) -> D/1
  Sum3/1 -> Saturation/1
  Saturation/1 -> yawRateCtrlOut/1

== system Leader/Ardupilot Attitude Controller/Attitude Controller/input_euler_angle_roll_pitch_euler_rate_yaw()/Add feedforward to angVelBody ==
  note: Thrust error angle above which yaw corrections are limited
  angVelBodyFeedforward : Inport
  angVelBodyIn : Inport  Port=2
  thurstErrorAngle : Inport  Port=3
  yawRateAct : Inport  Port=4
  ATC.THRUST_ERROR_ANGLE : Constant  Value=30.0
  MATLAB Function : MATLAB Function  TreatAsAtomicUnit=on
  deg to rad : Gain  Gain=pi/180
  angVelBody : Outport
  feedforwardScaler : Outport  Port=2
  wires:
  angVelBodyFeedforward/1 -> MATLAB Function/1(angVelBodyFeedforward)
  angVelBodyIn/1 -> MATLAB Function/2(angVelBodyIn)
  thurstErrorAngle/1 -> MATLAB Function/3(thrustErrorAngle)
  yawRateAct/1 -> MATLAB Function/4(yawRateAct)
  MATLAB Function/1(angVelBodyNew) -> angVelBody/1
  MATLAB Function/2(feedforwardScaler) -> feedforwardScaler/1
  ATC.THRUST_ERROR_ANGLE/1 -> deg to rad/1
  deg to rad/1 -> MATLAB Function/5(maxThrustErrorAngle4YawCorr)

== system Leader/Ardupilot Attitude Controller/Attitude Controller/input_euler_angle_roll_pitch_euler_rate_yaw()/Feedforward disabled ==
  note: QuaternionT<T>::from_euler()
      | Computes the quaternion from the given euler angles
  note: This subsystem represents to part of input_euler_angle_roll_pitch_euler_rate_yaw() that is executed, when the feedforward is disabled ( ATC_RATE_FF_ENAB = 0 )
  eulerAngleTar : Inport
  eulerInputDes : Inport  Port=2
  Constant : Constant  Value=0
  Constant1 : Constant  Value=0
  Demux : Demux  Outputs=3
  MATLAB Function : MATLAB Function  TreatAsAtomicUnit=on
  Selector : Selector  InputPortWidth=3  IndexOptions=Index vector (dialog)  Indices=[3]  OutputSizes=1
  Sum : Sum  Inputs=|++
  dt : Gain  Gain=0.01
  eulerRateTar : Outport
  angVelTar : Outport  Port=2
  attitudeTarget : Outport  Port=3
  wires:
  MATLAB Function/1(q) -> attitudeTarget/1  "attitudeTarget"
  Demux/1 -> MATLAB Function/1(roll)
  Demux/2 -> MATLAB Function/2(pitch)
  eulerInputDes/1 -> Demux/1
  Demux/3 -> dt/1
  dt/1 -> Sum/1
  Sum/1 -> MATLAB Function/3(yaw)
  eulerAngleTar/1 -> Selector/1
  Constant/1 -> eulerRateTar/1
  Constant1/1 -> angVelTar/1
  Selector/1 -> Sum/2

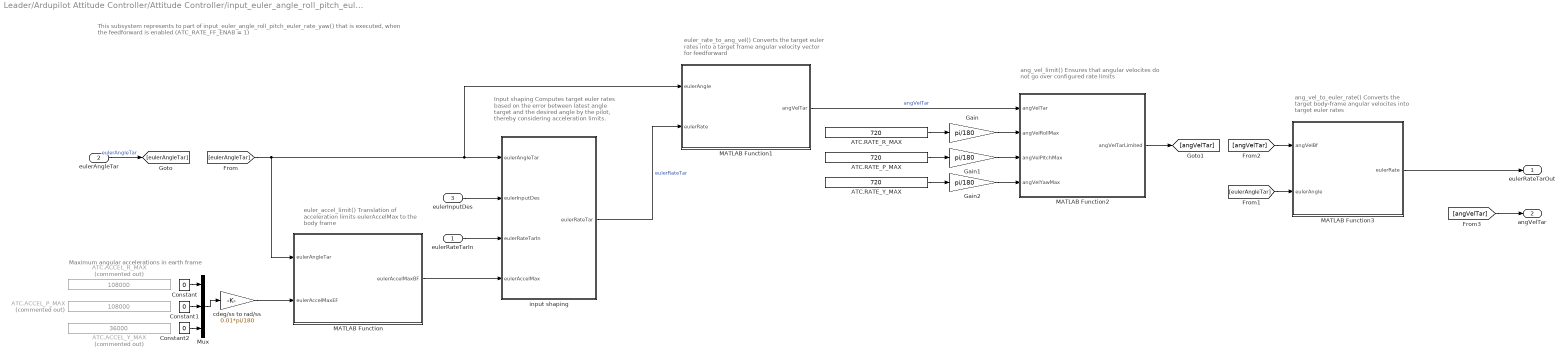
== system Leader/Ardupilot Attitude Controller/Attitude Controller/input_euler_angle_roll_pitch_euler_rate_yaw()/Feedforward enabled ==
  note: euler_rate_to_ang_vel()
      | Converts the target euler rates into a target frame angular velocity vector for feedforward
  note: euler_accel_limit()
      | Translation of acceleration limits eulerAccelMax to the body frame
  note: This subsystem represents to part of input_euler_angle_roll_pitch_euler_rate_yaw() that is executed, when the feedforward is enabled (ATC_RATE_FF_ENAB = 1)
  note: Maximum angular accelerations in earth frame
  note: Input shaping
      | Computes target euler rates based on the error between latest angle target and the desired angle by the pilot, thereby considering acceleration limits.
  note: ang_vel_limit()
      | Ensures that angular velocites do not go over configured rate limits
  note: ang_vel_to_euler_rate()
      | Converts the target body-frame angular velocites into target euler rates
  eulerRateTarIn : Inport
  eulerAngleTar : Inport  Port=2
  eulerInputDes : Inport  Port=3
  ATC.ACCEL_P_MAX : Constant  Commented=on  Value=108000
  ATC.ACCEL_R_MAX : Constant  Commented=on  Value=108000
  ATC.ACCEL_Y_MAX : Constant  Commented=on  Value=36000
  ATC.RATE_P_MAX : Constant  Value=720
  ATC.RATE_R_MAX : Constant  Value=720
  ATC.RATE_Y_MAX : Constant  Value=720
  Constant : Constant  Value=0
  Constant1 : Constant  Value=0
  Constant2 : Constant  Value=0
  Gain : Gain  Gain=pi/180
  Gain1 : Gain  Gain=pi/180
  Gain2 : Gain  Gain=pi/180
  MATLAB Function : MATLAB Function  TreatAsAtomicUnit=on
  MATLAB Function1 : MATLAB Function  TreatAsAtomicUnit=on
  MATLAB Function2 : MATLAB Function  TreatAsAtomicUnit=on
  MATLAB Function3 : MATLAB Function  TreatAsAtomicUnit=on
  Mux : Mux  Inputs=3
  cdeg/ss to rad/ss : Gain  Gain=0.01*pi/180
  input shaping : Subsystem
  eulerRateTarOut : Outport
  angVelTar : Outport  Port=2
  wires:
  [eulerAngleTar] -> MATLAB Function/1(eulerAngleTar), MATLAB Function1/1(eulerAngle), input shaping/1(eulerAngleTar)
  Mux/1 -> cdeg/ss to rad/ss/1
  MATLAB Function/1(eulerAccelMaxBF) -> input shaping/4(eulerAccelMax)
  eulerInputDes/1 -> input shaping/2(eulerInputDes)
  eulerRateTarIn/1 -> input shaping/3(eulerRateTarIn)
  input shaping/1(eulerRateTar) -> MATLAB Function1/2(eulerRate)  "eulerRateTar"
  MATLAB Function1/1(angVelTar) -> MATLAB Function2/1(angVelTar)  "angVelTar"
  Gain/1 -> MATLAB Function2/2(angVelRollMax)
  ATC.RATE_R_MAX/1 -> Gain/1
  ATC.RATE_P_MAX/1 -> Gain1/1
  Gain1/1 -> MATLAB Function2/3(angVelPitchMax)
  Gain2/1 -> MATLAB Function2/4(angVelYawMax)
  ATC.RATE_Y_MAX/1 -> Gain2/1
  eulerAngleTar/1 -> [eulerAngleTar]  "eulerAngleTar"
  [eulerAngleTar] -> MATLAB Function3/2(eulerAngle)
  MATLAB Function3/1(eulerRate) -> eulerRateTarOut/1
  MATLAB Function2/1(angVelTarLimited) -> [angVelTar]
  [angVelTar] -> MATLAB Function3/1(angVelBf)
  [angVelTar] -> angVelTar/1
  cdeg/ss to rad/ss/1 -> MATLAB Function/2(eulerAccelMaxEF)
  Constant1/1 -> Mux/2
  Constant/1 -> Mux/1
  Constant2/1 -> Mux/3

== system Leader/Ardupilot Attitude Controller/Attitude Controller/input_euler_angle_roll_pitch_euler_rate_yaw()/Update attitudeTarget ==
  note: Normalize attitudeTarget
  note: Use angVelTar to rotate attitudeTarget
  note: Use rotated attitudeTarget, if FF is enabled.
      | Otherwise, use unchanged attitudeTarget
  attitudeTarget : Inport
  angVelTar : Inport  Port=2
  ffEnabled : Inport  Port=3
  MATLAB Function : MATLAB Function  TreatAsAtomicUnit=on
  Rotate target attitude : Subsystem
  Switch : Switch  Criteria=u2 > Threshold  SaturateOnIntegerOverflow=off  InputSameDT=off
  attitudeTargetUpdate : Outport
  wires:
  MATLAB Function/1(qNorm) -> attitudeTargetUpdate/1
  Switch/1 -> MATLAB Function/1(q)
  ffEnabled/1 -> Switch/2
  attitudeTarget/1 -> Switch/3, Rotate target attitude/1(attitudeTarget)
  angVelTar/1 -> Rotate target attitude/2(angVelTar)
  Rotate target attitude/1(attitudeTargetRot) -> Switch/1

== system Leader/Ardupilot Attitude Controller/Attitude Controller/input_euler_angle_roll_pitch_euler_rate_yaw()/reset yaw targets ==
  note: "ahrs.yaw - euler_angle_target.z"
  note: This subsystem resets the yaw target angle and rate, if the throttle is zero, meaning that the copter is landed. The respective function is AC_AttitudeControl::reset_yaw_target_and_rate() , which is called in ModeStabilize::run() when the copter is armed, but throttle is still zero.
  eulerRateTarIn : Inport
  attitudeTargetIn : Inport  Port=2
  eulerAngleAct : Inport  Port=3
  throttle : Inport  Port=4
  Demux : Demux  Outputs=3
  Demux1 : Demux  Outputs=3
  MATLAB Function1 : MATLAB Function  TreatAsAtomicUnit=on
  MATLAB Function5 : MATLAB Function  TreatAsAtomicUnit=on
  MATLAB Function9 : MATLAB Function  TreatAsAtomicUnit=on
  Mux : Mux  Inputs=3
  Mux1 : Mux  Inputs=3
  Subtract : Sum  Inputs=-+
  Switch : Switch  Criteria=u2 > Threshold  SaturateOnIntegerOverflow=off  InputSameDT=off
  Switch1 : Switch  Criteria=u2 > Threshold  SaturateOnIntegerOverflow=off  InputSameDT=off
  Terminator{,1..4} (5 alike) : Terminator
  Zero : Constant  Value=0
  Zero1 : Constant  Value=0
  Zero2 : Constant  Value=0
  eulerRateTar : Outport
  attitudeTarget : Outport  Port=2
  wires:
  Switch1/1 -> attitudeTarget/1
  Switch/1 -> eulerRateTar/1
  throttle/1 -> Switch1/2, Switch/2
  eulerRateTarIn/1 -> Demux1/1, Switch/1
  eulerAngleAct/1 -> Demux/1
  MATLAB Function9/1(qRes) -> Switch1/3
  attitudeTargetIn/1 -> Switch1/1, MATLAB Function9/2(q2), MATLAB Function1/1(q)
  MATLAB Function1/3(yaw) -> Subtract/1  "yawAngleTar"
  MATLAB Function1/1(roll) -> Terminator/1
  MATLAB Function1/2(pitch) -> Terminator1/1
  Demux/1 -> Terminator2/1
  Demux/2 -> Terminator3/1
  Demux/3 -> Subtract/2
  Subtract/1 -> Mux/3
  MATLAB Function5/1(q) -> MATLAB Function9/1(q1)  "attitudeTargetUpdate"
  Mux/1 -> MATLAB Function5/1(vec)
  Zero/1 -> Mux/1
  Zero1/1 -> Mux/2
  Mux1/1 -> Switch/3
  Demux1/1 -> Mux1/1
  Demux1/2 -> Mux1/2
  Demux1/3 -> Terminator4/1
  Zero2/1 -> Mux1/3

== system Leader/Ardupilot Attitude Controller/Attitude Controller/input_euler_angle_roll_pitch_euler_rate_yaw()/thrust_heading_rotation_angles() ==
  note: Limit yaw error based in maximum acceleration
  note: AC_AttitudeControl::thrust_vector_rotation_angles()
      | Calculation of thrust_angle, thrust_error_angle, attitude_error and thrust_vector_correction
  note: This subsystem contains all the calculations contained in the function AC_AttitudeControl::thrust_heading_rotation_angles() that is called in AC_AttitudeControl::attitude_controller_run_quat()
  attitudeTargetIn : Inport
  attitudeBodyAct : Inport  Port=2
  Yaw error limitation : Subsystem
  thrust_vector_rotation_angles() : Subsystem
  attitudeTarget : Outport
  attitudeError : Outport  Port=2
  thrustErrorAngle : Outport  Port=3
  thrustAngle : Outport  Port=4
  wires:
  attitudeTargetIn/1 -> [attitudeTarget]  "attTar"
  [attitudeBody] -> thrust_vector_rotation_angles()/2(attitudeBodyAct)
  thrust_vector_rotation_angles()/1(attitudeError) -> Yaw error limitation/1(attitudeErrorIn)
  thrust_vector_rotation_angles()/3(thrustErrAngle) -> thrustErrorAngle/1
  thrust_vector_rotation_angles()/2(thrustVecCorrection) -> Yaw error limitation/2(thrustVecCorrection)
  thrust_vector_rotation_angles()/4(thrustAngle) -> thrustAngle/1
  attitudeBodyAct/1 -> [attitudeBody]  "attBody"
  [attitudeBody] -> Yaw error limitation/3(attitudeBody)
  Yaw error limitation/1(atitudeTarget) -> attitudeTarget/1
  Yaw error limitation/2(attitudeError) -> attitudeError/1
  [attitudeTarget] -> thrust_vector_rotation_angles()/1(attitudeTarget)
  [attitudeTarget] -> Yaw error limitation/4(attitudeTarget)

== system Leader/Ardupilot Attitude Controller/Attitude Controller/input_euler_angle_roll_pitch_euler_rate_yaw()/update_ang_vel_target_from_att_error() ==
  note: The subsystems either use the square root controller or an easy proportional relation (kp*err) to calculate the target angular velocity
  note: AC_AttitudeControl::update_ang_vel_target_from_att_error()
      | Compute the angular velocity corrections in the body frame from the attitude error.
  attitudeError : Inport
  Calc angular velocity target pitch : Subsystem
  Calc angular velocity target roll : Subsystem
  Calc angular velocity target yaw : Subsystem
  Mux : Mux  Inputs=3
  Scope : Scope  NumInputPorts=3
  Selector : Selector  InputPortWidth=3  IndexOptions=Index vector (dialog)  Indices=[1]  OutputSizes=1
  Selector1 : Selector  InputPortWidth=3  IndexOptions=Index vector (dialog)  Indices=[2]  OutputSizes=1
  Selector2 : Selector  InputPortWidth=3  IndexOptions=Index vector (dialog)  Indices=[3]  OutputSizes=1
  angVelBody : Outport
  wires:
  attitudeError/1 -> Selector2/1, Selector/1, Selector1/1
  Mux/1 -> angVelBody/1
  Selector/1 -> Scope/1, Calc angular velocity target roll/1(attitudeErrorRoll)
  Calc angular velocity target roll/1(angVelRoll) -> Mux/1
  Calc angular velocity target yaw/1(angVelYaw) -> Mux/3
  Calc angular velocity target pitch/1(angVelPitch) -> Mux/2
  Selector2/1 -> Scope/3, Calc angular velocity target yaw/1(attitudeErrorYaw)
  Selector1/1 -> Scope/2, Calc angular velocity target pitch/1(attitudeErrorPitch)

== system Leader/Ardupilot Attitude Controller/Rate Controller/PID Pitch Rate/Calc Derivative ==
  e : Inport
  ATC Sampling Time : Constant  Value=0.01
  Divide : Product  Inputs=*/
  Sum : Sum  Inputs=|+-  OutDataTypeStr=double
  Unit Delay : UnitDelay  SampleTime=-1  HasFrameUpgradeWarning=on
  derivative : Outport
  wires:
  e/1 -> Sum/1, Unit Delay/1
  Unit Delay/1 -> Sum/2
  Sum/1 -> Divide/1
  Divide/1 -> derivative/1
  ATC Sampling Time/1 -> Divide/2

== system Leader/Ardupilot Attitude Controller/Rate Controller/PID Pitch Rate/I ==
  note: Integrator, see AC_PID::update_i()
  e : Inport
  limitFlg : Inport  Port=2
  ki : Inport  Port=3
  i_max : Inport  Port=4
  ATC Sampling Time : Constant  Value=0.01
  Cast To Double : DataTypeConversion  OutDataTypeStr=double  SaturateOnIntegerOverflow=off  RndMeth=Floor
  Integrator : MATLAB Function  TreatAsAtomicUnit=on
  Unit Delay : UnitDelay  SampleTime=-1  HasFrameUpgradeWarning=on
  integrator : Outport
  wires:
  [integrator_out] -> integrator/1
  ki/1 -> Integrator/4(ki)
  i_max/1 -> Integrator/5(i_max)
  e/1 -> Integrator/1(error)
  ATC Sampling Time/1 -> Integrator/6(dt)
  limitFlg/1 -> Integrator/3(limit_flg)
  Integrator/1(integrator_out) -> Cast To Double/1
  Cast To Double/1 -> [integrator_out]
  [integrator_out] -> Unit Delay/1
  Unit Delay/1 -> Integrator/2(integrator)

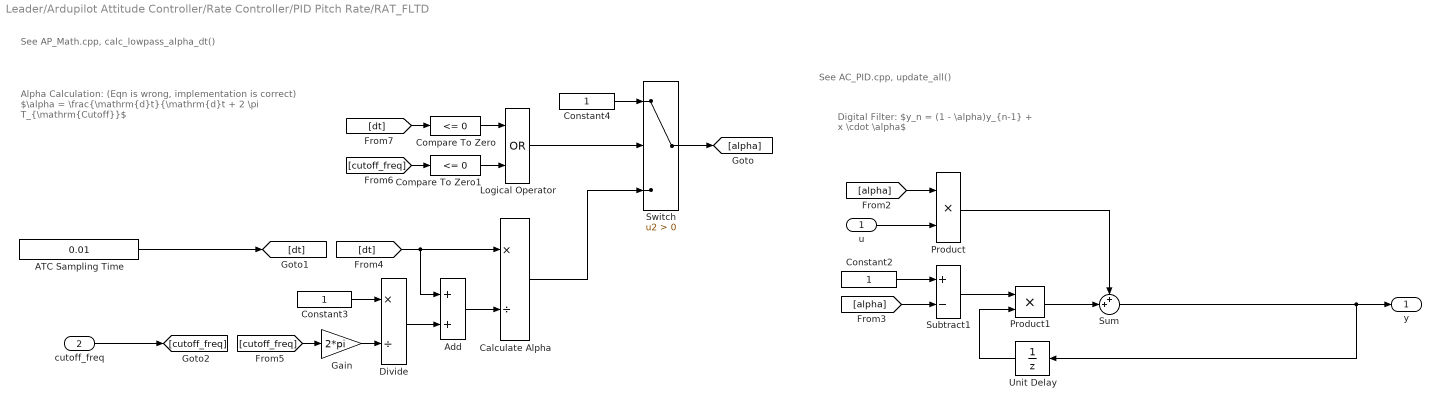
== system Leader/Ardupilot Attitude Controller/Rate Controller/PID Pitch Rate/RAT_FLTD ==
  note: Digital Filter:
      | $y_n = (1 - \alpha)y_{n-1} + x \cdot \alpha$
  note: See AC_PID.cpp, update_all()
  note: See AP_Math.cpp, calc_lowpass_alpha_dt()
  note: Alpha Calculation: (Eqn is wrong, implementation is correct)
      | $\alpha = \frac{\mathrm{d}t}{\mathrm{d}t + 2 \pi T_{\mathrm{Cutoff}}$
  u : Inport
  cutoff_freq : Inport  Port=2
  ATC Sampling Time : Constant  Value=0.01
  Add : Sum
  Calculate Alpha : Product  Inputs=*/
  Compare To Zero : simulink/Logic and Bit Operations/Compare To Zero  relop=<=  OutDataTypeStr=boolean
  Compare To Zero1 : simulink/Logic and Bit Operations/Compare To Zero  relop=<=  OutDataTypeStr=boolean
  Constant2 : Constant
  Constant3 : Constant
  Constant4 : Constant
  Divide : Product  Inputs=*/
  Gain : Gain  Gain=2*pi
  Logical Operator : Logic  Operator=OR  AllPortsSameDT=off  OutDataTypeStr=boolean
  Product : Product
  Product1 : Product
  Subtract1 : Sum  Inputs=+-
  Sum : Sum  Inputs=++|  OutDataTypeStr=double  AccumDataTypeStr=double
  Switch : Switch  Criteria=u2 > Threshold  SaturateOnIntegerOverflow=off  InputSameDT=off
  Unit Delay : UnitDelay  SampleTime=-1  HasFrameUpgradeWarning=on
  y : Outport
  wires:
  Product1/1 -> Sum/2
  Unit Delay/1 -> Product1/2
  Subtract1/1 -> Product1/1
  [alpha] -> Subtract1/2
  Constant2/1 -> Subtract1/1
  [alpha] -> Product/1
  Calculate Alpha/1 -> Switch/3
  Add/1 -> Calculate Alpha/2
  [dt] -> Add/1, Calculate Alpha/1
  Gain/1 -> Divide/2
  cutoff_freq/1 -> [cutoff_freq]
  u/1 -> Product/2
  Divide/1 -> Add/2
  Constant3/1 -> Divide/1
  Product/1 -> Sum/1
  Switch/1 -> [alpha]
  [cutoff_freq] -> Gain/1
  [dt] -> Compare To Zero/1
  [cutoff_freq] -> Compare To Zero1/1
  Compare To Zero/1 -> Logical Operator/1
  Compare To Zero1/1 -> Logical Operator/2
  Logical Operator/1 -> Switch/2
  Constant4/1 -> Switch/1
  Sum/1 -> Unit Delay/1, y/1
  ATC Sampling Time/1 -> [dt]

== system Leader/Ardupilot Attitude Controller/Rate Controller/PID Pitch Rate/RAT_FLTE ==
  note: Digital Filter:
      | $y_n = (1 - \alpha)y_{n-1} + x \cdot \alpha$
  note: See AC_PID.cpp, update_all()
  note: See AP_Math.cpp, calc_lowpass_alpha_dt()
  note: Alpha Calculation: (Eqn is wrong, implementation is correct)
      | $\alpha = \frac{\mathrm{d}t}{\mathrm{d}t + 2 \pi T_{\mathrm{Cutoff}}$
  u : Inport
  cutoff_freq : Inport  Port=2
  ATC Sampling Time : Constant  Value=0.01
  Add : Sum
  Calculate Alpha : Product  Inputs=*/
  Compare To Zero : simulink/Logic and Bit Operations/Compare To Zero  relop=<=  OutDataTypeStr=boolean
  Compare To Zero1 : simulink/Logic and Bit Operations/Compare To Zero  relop=<=  OutDataTypeStr=boolean
  Constant2 : Constant
  Constant3 : Constant
  Constant4 : Constant
  Divide : Product  Inputs=*/
  Gain : Gain  Gain=2*pi
  Logical Operator : Logic  Operator=OR  AllPortsSameDT=off  OutDataTypeStr=boolean
  Product : Product
  Product1 : Product
  Subtract1 : Sum  Inputs=+-
  Sum : Sum  Inputs=++|  OutDataTypeStr=double
  Switch : Switch  Criteria=u2 > Threshold  SaturateOnIntegerOverflow=off  InputSameDT=off
  Unit Delay : UnitDelay  SampleTime=-1  HasFrameUpgradeWarning=on
  y : Outport
  wires:
  Product1/1 -> Sum/2
  Unit Delay/1 -> Product1/2
  Subtract1/1 -> Product1/1
  [alpha] -> Subtract1/2
  Constant2/1 -> Subtract1/1
  [alpha] -> Product/1
  Calculate Alpha/1 -> Switch/3
  Add/1 -> Calculate Alpha/2
  [dt] -> Add/1, Calculate Alpha/1
  cutoff_freq/1 -> [cutoff_freq]
  u/1 -> Product/2
  Product/1 -> Sum/1
  Switch/1 -> [alpha]
  [dt] -> Compare To Zero/1
  [cutoff_freq] -> Compare To Zero1/1
  Compare To Zero/1 -> Logical Operator/1
  Compare To Zero1/1 -> Logical Operator/2
  Logical Operator/1 -> Switch/2
  Constant4/1 -> Switch/1
  Sum/1 -> Unit Delay/1, y/1
  ATC Sampling Time/1 -> [dt]
  [cutoff_freq] -> Gain/1
  Divide/1 -> Add/2
  Constant3/1 -> Divide/1
  Gain/1 -> Divide/2
